simulink model "example_NMPC_BGLOSA_redTh_V500_platoon"  (R2022b)
settings: Solver=ode4  StartTime=0.0  StopTime=1500  FixedStep=0.1  RelTol=1e-3
PostLoadFcn:
  | , if any(exist('dsrtsu_mdlpostloadfcn', 'file') == [2, 3, 6]), try dsrtsu_mdlpostloadfcn('Execute', bdroot); catch fprintf('Error in PostLoadFcn (dsrtsu_mdlpostloadfcn) for model "%s":\n %s\n', bdroot, lasterr); end, end,
values from neighbouring files (symbols this model uses):
  k_road_map = k_road_map(:)    [NMPC_init.m]
  N = 50    [ACADO_BGLOSA_soft_constraints_platoon.m]    (also in ACADO_BGLOSA_soft_constraints_platoon_stop_dwell.m; NMPC_init.m)
  N_iter = 3    [NMPC_init.m]
  N_Jterms = length(Qx1)    [NMPC_init.m]
  NMPC_Wmat1 = [W1(1,:) W1(2,:) W1(3,:) W1(4,:) W1(5,:) W1(6,:) W1(7,:) W1(8,:) W1(9,:)]    [NMPC_init.m]
  NMPC_WNmat1 = reshape(WN1.',1,[])    [NMPC_init.m]
  t_dwell = 10    [ACADO_BGLOSA_soft_constraints_platoon.m]    (also in ACADO_BGLOSA_soft_constraints_platoon_stop_dwell.m; NMPC_init.m)
  t_offset = 0    [NMPC_init.m]
  time_bag_sim = (0:1:round(time_bag(end))-1)'    [NMPC_init.m]
  tl_state_sim = zeros(round(time_bag(end))-1,size(tl_col,2))    [NMPC_init.m]
  Ts = 1    [ACADO_BGLOSA_soft_constraints_platoon.m]    (also in ACADO_BGLOSA_soft_constraints_platoon_stop_dwell.m; NMPC_init.m)
  Vmax = 50    [NMPC_init.m]
  xInit = [0 2 0]    [NMPC_init.m]
undefined symbols (not defined in the file or in its folder): ds, s_start
libraries: simulink x1
(part 1 of 2)
settings Model: DSRTSU_INTERNAL_RTI_VER=450  DSRTSU_INTERNAL_RTI_TYPE=rti1401  DSRTSU_INTERNAL_RTIFPGA=40  Creator=d068515  LastModifiedBy=ricca
settings DataIOCC: SaveFormat=StructureWithTime
settings OptimizationCC: BlockReduction=off  LifeSpan=inf
settings DebuggingCC: SFExecutionAtInitializationDiag=none  SFMachineParentedDataDiag=warning  ArithmeticOperatorsInVariantConditions=warning
settings HardwareCC: ProdBitPerSizeT=32  ProdBitPerPtrDiffT=32  ProdEndianess=BigEndian  ProdWordSize=32  ProdHWDeviceType=Generic->Custom  TargetIntDivRoundTo=Zero  TargetEndianess=BigEndian  TargetHWDeviceType=Generic->Custom
settings SFSimCC: CustomCodeUndefinedFunction=UseInterfaceOnly
settings RTWCC: Description=dSPACE DS1401 Hardware Platform  SystemTargetFile=rti1401.tlc  MakeCommand=make_rti  TemplateMakefile=rti1401.tmf
settings CodeAppCC: StateflowObjectComments=on
settings STFCustomTargetCC: ParMdlRefBuildCompliant=on  GRTInterface=on  SystemTargetFile=rti1401.tlc
settings GRTTargetCC: TargetLangStandard=C89/C90 (ANSI)  CompOptLevelCompliant=off  ConcurrentExecutionCompliant=off  CombineOutputUpdateFcns=off  MatFileLogging=off  CPPClassGenCompliant=off  GRTInterface=on  UseToolchainInfoCompliant=off  ExtModeMexFile=noextcomm

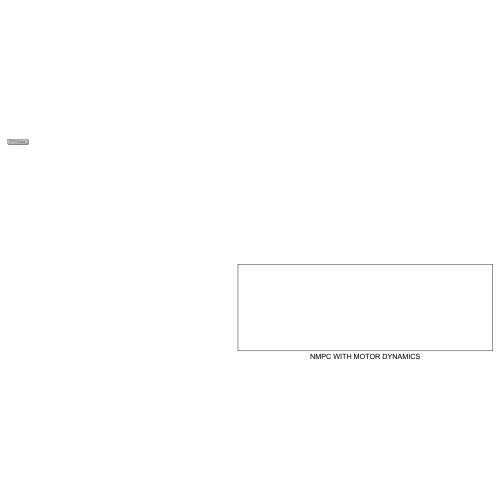
[thumbnail: Simulink's stored preview of the top-level diagram]
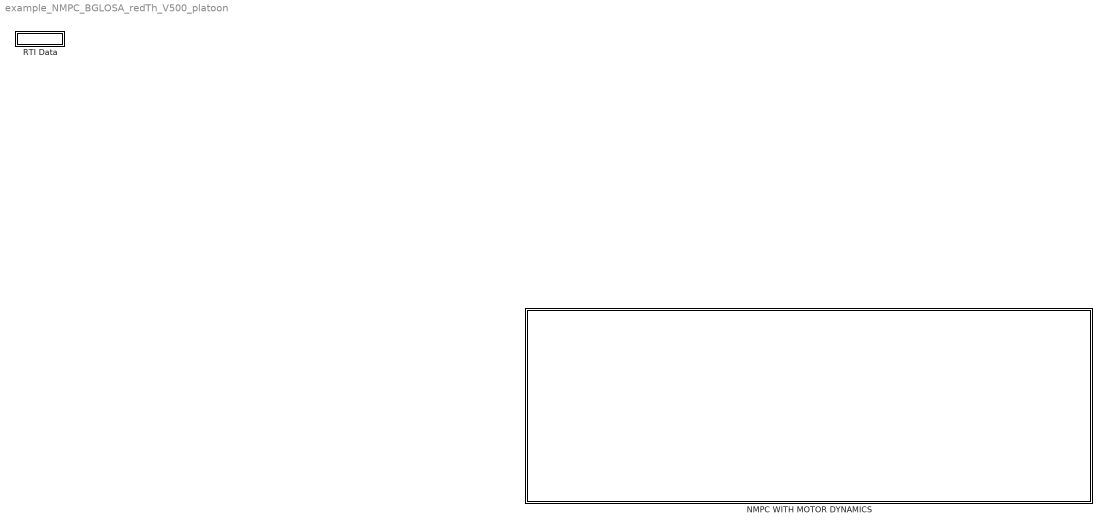
== system example_NMPC_BGLOSA_redTh_V500_platoon ==
  NMPC WITH MOTOR DYNAMICS : Subsystem
  RTI Data : Subsystem  Tag=struct('RTIDataServer',struct('RTIDataServerVs','2','RTIModelDescription','struct(''main'',''TC_RAF_2014b'',''sub'','''',''isMp'',0)'))  LoadFcn="if exist('rtidc'), try,  rtidc('DataHostBlockClbLoad', gcbh); catch, disp(['Warning: ''LoadFcn'' for RTI Data block failed: ' lasterr]); end, end,"  mask(RTI_DATA_HOST){}
      mask help:
      | RTI Data Block.
      | This block is used by RTI to store internal model-dependent data.
      | Please keep this block on the root level of the model. Deleting this block will result in data loss.
      |
      | NEVER DELETE OR COPY THIS BLOCK!
      settings: CopyFcn="if exist('rtidc'), try,  rtidc('DataHostBlockClbCopy', gcbh); catch, disp(['Warning: ''CopyFcn'' for RTI Data block failed: ' lasterr]); end, end,"  DeleteFcn="if exist('rtidc'), try,  rtidc('DataHostBlockClbDelete', gcbh); catch, disp(['Warning: ''DeleteFcn'' for RTI Data block failed: ' lasterr]); end, end,"  ModelCloseFcn="if exist('rtidc'), try,  rtidc('DataHostBlockClbModelClose', gcbh); catch, disp(['Warning: ''ModelCloseFcn'' for RTI Data block failed: ' lasterr]); end, end,"  PreSaveFcn="if exist('rtidc'), try,  rtidc('DataHostBlockClbPreSave', gcbh); catch, disp(['Warning: ''PreSaveFcn'' for RTI Data block failed: ' lasterr]); end, end,"  PostSaveFcn="if exist('rtidc'), try,  rtidc('DataHostBlockClbPostSave', gcbh); catch, disp(['Warning: ''PostSaveFcn'' for RTI Data block failed: ' lasterr]); end, end,"  NameChangeFcn="if exist('rtidc'), try,  rtidc('DataHostBlockClbNameChange', gcbh); catch, disp(['Warning: ''NameChangeFcn'' for RTI Data block failed: ' lasterr]); end, end,"
      mask Help:
      | RTI Data Block.
      | This block is used by RTI to store internal model-dependent data.
      | Please keep this block on the root level of the model. Deleting this block will result in data loss.
      | 
      | NEVER DELETE OR COPY THIS BLOCK!
      mask Display:
      | text(0.5, 0.5, 'RTI Data', 'HorizontalAlignment', 'center');
      | plot([1 0]);

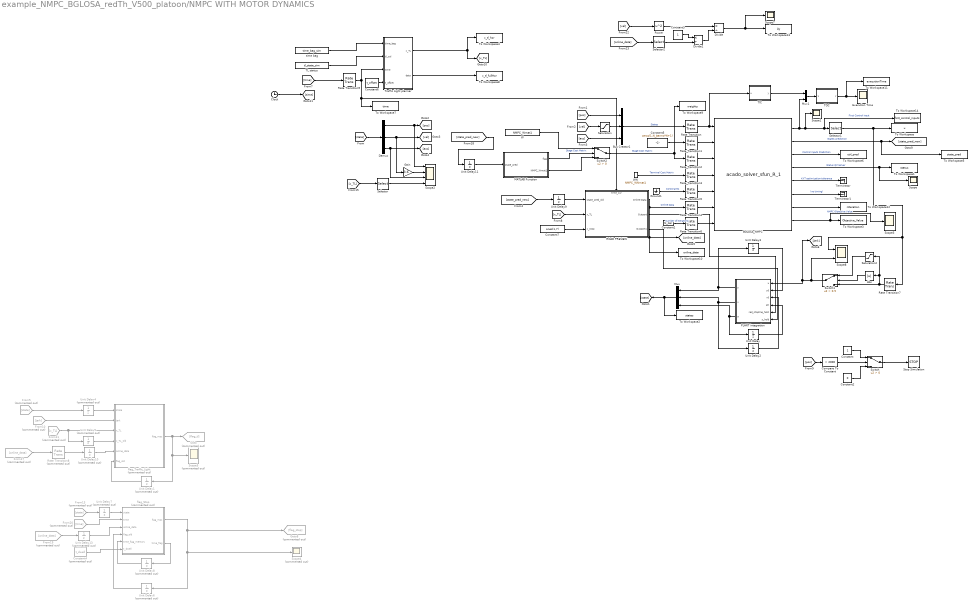
== system example_NMPC_BGLOSA_redTh_V500_platoon/NMPC WITH MOTOR DYNAMICS ==
  Abs : Abs  SaturateOnIntegerOverflow=off
  BGLOSA_NMPC : S-Function  FunctionName=acado_solver_sfun_R_1  Parameters=xInit, zInit, uInit, NMPC_Wmat1, NMPC_WNmat1, bValues  SFunctionDeploymentMode=off  EnableBusSupport=off  mask(Legacy Function){SFunctionSpec=acado_step(ACADOinput u1[1], ACADOoutput y1[1]), ShowSpec=on}
      mask prompts: ShowSpec "Display function specification"
      mask help:
      | This block allows you to call the legacy functions specified by the following Legacy Code Tool definition:
      | def.SFunctionName = 'acado_solver_sfun';
      | def.OutputFcnSpec = 'acado_step(ACADOinput u1[1], ACADOoutput y1[1])';
      | def.StartFcnSpec = 'acado_initialize( void )';
      | def.TerminateFcnSpec = 'acado_cleanup( void )';
      | def.HeaderFiles = {'acado_common.h', 'acado_solver_sfunction.h'};
      | def.SourceFiles = {'acado_solver.c', 'acado_integrator.c', 'acado_auxiliary_functions.c', 'acado_solver_sfunction.c', 'acado_qpoases_interface.cpp', 'qpoases/SRC/Bounds.cpp', 'qpoases/SRC/Constraints.cpp', 'qpoases/SRC/CyclingManager.cpp', 'qpoases/SRC/Indexlist.cpp', 'qpoases/SRC/MessageHandling.cpp', 'qpoases/SRC/QProblem.cpp', 'qpoases/SRC/QProblemB.cpp', 'qpoases/SRC/SubjectTo.cpp', 'qpoases/SRC/Utils.cpp', 'qpoases/SRC/EXTRAS/SolutionAnalysis.cpp'};
      | def.IncPaths = {'qpoases', 'qpoases/INCLUDE', 'qpoases/SRC'};
      | def.Options.language = 'C++';
      mask Help: <p>This block was generated automatically by the Legacy Code Tool. For detailed help on this tool, call<a href="matlab:legacy_code('help')"> legacy_code('help')</a>.</p>
      mask Callback ShowSpec:
      | if strcmp(get_param(gcbh, 'ShowSpec'), 'on')
      |   set_param(gcbh, 'MaskDisplay', sprintf('fprintf(''%s'');', get_param(gcbh, 'SFunctionSpec')));
      | else
      |   set_param(gcbh, 'MaskDisplay', sprintf('fprintf(''%s'');', get_param(gcbh, 'FunctionName')));
      | end
      mask Display: fprintf('acado_step(ACADOinput u1[1], ACADOoutput y1[1])');
  Bus Creator1 : BusCreator  Inputs=3
  Clock : Clock
  Compare To Constant : simulink/Logic and Bit Operations/Compare To Constant  relop=>  const=2000  OutDataTypeStr=boolean
  Constant : Constant
  Constant1 : Constant  Value=N_iter
  Constant2 : Constant  Value=0
  Constant3 : Constant
  Constant4 : Constant  Commented=on  Value=t_dwell
  Constant5 : Constant  Value=zeros(1,N_Jterms*N+1)
  Constant6 : Constant  Value=t_offset
  Constant7 : Constant  Value=ones(1,7)
  Demux : Demux  Outputs=3
  Divide : Product  Inputs=*/
  Divide1 : Product  Inputs=*/
  Execution Time : Scope
  From10 : From  Commented=on  GotoTag=jerk
  From11 : From  Commented=on  GotoTag=x_TL
  From13 : From  Commented=on  GotoTag=state
  From17 : From  Commented=on  GotoTag=online_data
  From19 : From  Commented=on  GotoTag=online_data
  From20 : From  Commented=on  GotoTag=time
  From5 : From  Commented=on  GotoTag=state
  Gain : Gain  Gain=3.6
  Goto : Goto  Commented=on  GotoTag=flag_tl
  Goto8 : Goto  Commented=on  GotoTag=flag_stop
  Ground1 : Ground
  MATLAB Function : MATLAB Function  TreatAsAtomicUnit=on
  Mux : Mux  Inputs=3
  Mux1 : Mux  Inputs=2
  PLANT integration : MATLAB Function  TreatAsAtomicUnit=on
  Power : Math  Operator=square
  ROAD PREVIEW : Subsystem
      settings: PortSchema="{\"entries\":[{\"content\":{\"sides\":[{\"content\":{\"connectorIds\":[\"In1\",\"In2\",\"In3\"]},\"type\":\"ConnectorPlacement.EquallySpacedRectSide\",\"uuid\":\"89746bc5-bd2f-4e61-9556-28242176c46a\"},{\"content\":{\"connectorIds\":[\"Out1\",\"Out2\",\"Out3\"],\"side\":\"RIGHT\"},\"type\":\"ConnectorPlacement.EquallySpacedRectSide\",\"uuid\":\"fa5eae8e-eb55-42b4-8d8b-02c8b36cc91d\"},{\"content\":{\"connectorIds\":[\"In4\"],\"side\":\"TOP\"},\"type\":\"ConnectorPlacement.EquallySpacedRectSide\",\"uuid\":\"5942e98b-dfb5-4e56-acd3-edfb2315bb7f\"}]},\"type\":\"ConnectorPlacement.EquallySpacedConnector\",\"uuid\":\"ba8f73d0-227f-4198-ac0b-e11b2a073141\"}],\"packageUris\":[\"http://schema.mathworks.com/mf0/Connector/R2020b\"],\"version\":\"1.0\"}"
  Rate Transition : RateTransition  Deterministic=off  InitialCondition=xInit  OutPortSampleTime=Ts
  Rate Transition{1..6} (6 alike) : RateTransition  Deterministic=off  OutPortSampleTime=Ts
  Rate Transition7 : RateTransition  Deterministic=off  OutPortSampleTime=0.1
  Rate Transition8 : RateTransition  Commented=on  InitialCondition=zeros(1665,1)  OutPortSampleTime=Ts
  Rate Transition9 : RateTransition  OutPortSampleTime=Ts
  Saturation : Saturate  UpperLimit=50/3.6  LowerLimit=0
  Saturation2 : Saturate  UpperLimit=0.1  LowerLimit=-0.1
  Scope{,1,3,7} (4 alike) : Scope
  Scope2 : Scope  NumInputPorts=4
  Scope4 : Scope  Commented=on
  Scope5 : Scope  Commented=on
  Scope8 : Scope  NumInputPorts=2
  Selector : Selector  NumberOfDimensions=2  InputPortWidth=3  IndexOptions=Index vector (dialog),Select all  Indices=1,1  OutputSizes=1,1
  Selector1 : Selector  InputPortWidth=3  IndexOptions=Index vector (dialog)  Indices=[1]  OutputSizes=1
  Selector2 : Selector  NumberOfDimensions=2  InputPortWidth=3  IndexOptions=Select all,Select all  Indices=28,1  OutputSizes=1,1
  Stop Simulation : Stop
  Switch : Switch  Criteria=u2 > Threshold  SaturateOnIntegerOverflow=off  InputSameDT=off
  Switch1 : Switch  Criteria=u2 > Threshold  Threshold=0.5  SaturateOnIntegerOverflow=off  InputSameDT=off
  Switch2 : Switch  Criteria=u2 > Threshold  SaturateOnIntegerOverflow=off  InputSameDT=off
  TIC : MATLAB Function  TreatAsAtomicUnit=on
  TL status : Constant  Value=tl_state_sim  OutDataTypeStr=double
  TOC : MATLAB Function  TreatAsAtomicUnit=on
  Terminator : Terminator
  Terminator1 : Terminator
  To Workspace : ToWorkspace  VariableName=u  SaveFormat=Structure With Time  SampleTime=-1
  To Workspace1 : ToWorkspace  VariableName=status  SaveFormat=Structure With Time  SampleTime=-1
  To Workspace10 : ToWorkspace  VariableName=online_data  SaveFormat=Structure With Time  SampleTime=-1
  To Workspace11 : ToWorkspace  VariableName=executionTime  SaveFormat=Structure With Time  SampleTime=-1
  To Workspace12 : ToWorkspace  VariableName=nIteration  SaveFormat=Structure With Time  SampleTime=-1
  To Workspace13 : ToWorkspace  VariableName=Ay  SaveFormat=Structure With Time  SampleTime=-1
  To Workspace14 : ToWorkspace  VariableName=first_control_inputs  SaveFormat=Timeseries  SampleTime=-1
  To Workspace2 : ToWorkspace  VariableName=states  SaveFormat=Structure With Time  SampleTime=-1
  To Workspace3 : ToWorkspace  VariableName=Objective_Value  SaveFormat=Structure With Time  SampleTime=-1
  To Workspace4 : ToWorkspace  VariableName=x_tl_hor  SaveFormat=Structure With Time  SampleTime=-1
  To Workspace5 : ToWorkspace  VariableName=state_pred  SaveFormat=Structure With Time  SampleTime=-1
  To Workspace6 : ToWorkspace  VariableName=ctrl_pred  SaveFormat=Structure With Time  SampleTime=-1
  To Workspace7 : ToWorkspace  VariableName=time  SaveFormat=Structure With Time  SampleTime=-1
  To Workspace8 : ToWorkspace  VariableName=x_tl_fullHor  SaveFormat=Structure With Time  SampleTime=-1
  To Workspace9 : ToWorkspace  VariableName=weights  SaveFormat=Structure With Time  SampleTime=-1
  Traffic Light planner : MATLAB Function  TreatAsAtomicUnit=on
  Unit Delay : UnitDelay  InitialCondition=xInit(3)  SampleTime=-1  HasFrameUpgradeWarning=on
  Unit Delay1 : UnitDelay  Commented=on  InitialCondition=zeros(1,11)  SampleTime=-1  HasFrameUpgradeWarning=on
  Unit Delay10 : UnitDelay  Commented=on  InitialCondition=zeros(50*(N+1),1)  SampleTime=-1  HasFrameUpgradeWarning=on
  Unit Delay11 : UnitDelay  InitialCondition=xInit.*ones(N+1,3)  SampleTime=-1  HasFrameUpgradeWarning=on
  Unit Delay13 : UnitDelay  Commented=on  InitialCondition=zeros(50*(N+1),1)  SampleTime=-1  HasFrameUpgradeWarning=on
  Unit Delay2 : UnitDelay  InitialCondition=xInit(2)  SampleTime=-1  HasFrameUpgradeWarning=on
  Unit Delay3 : UnitDelay  InitialCondition=xInit(1)  SampleTime=-1  HasFrameUpgradeWarning=on
  Unit Delay4 : UnitDelay  Commented=on  InitialCondition=xInit  SampleTime=-1  HasFrameUpgradeWarning=on
  Unit Delay5 : UnitDelay  Commented=on  InitialCondition=zeros(N+1,12)  SampleTime=-1  HasFrameUpgradeWarning=on
  Unit Delay6 : UnitDelay  Commented=on  InitialCondition=zeros(1,7)  SampleTime=-1  HasFrameUpgradeWarning=on
  Unit Delay7 : UnitDelay  Commented=on  InitialCondition=xInit  SampleTime=-1  HasFrameUpgradeWarning=on
  Unit Delay8 : UnitDelay  Commented=on  InitialCondition=zeros(1,7)  SampleTime=-1  HasFrameUpgradeWarning=on
  Unit Delay9 : UnitDelay  InitialCondition=xInit.*ones(N+1,3)  SampleTime=-1  HasFrameUpgradeWarning=on
  W : Constant  Value=NMPC_Wmat1  OutDataTypeStr=double
  "WN " : Constant  Value=NMPC_WNmat1  OutDataTypeStr=double
  flag_Stop : MATLAB Function  Commented=on  TreatAsAtomicUnit=on
  flag_Traffic_Light : MATLAB Function  Commented=on  TreatAsAtomicUnit=on
  time bag : Constant  Value=time_bag_sim  OutDataTypeStr=double
  wires:
  BGLOSA_NMPC/3 -> To Workspace6/1  "Control Inputs Prediction"
  BGLOSA_NMPC/4 -> To Workspace1/1, Scope/1  "Status QP Solver"
  Constant1/1 -> Rate Transition6/1  "Number of iterations"
  BGLOSA_NMPC/8 -> Scope3/1, To Workspace3/1  "NMPC Objective Value"
  Bus Creator1/1 -> Rate Transition/1  "States"
  BGLOSA_NMPC/1 -> Mux1/2, To Workspace14/1, Selector1/1, Scope1/1  "First Control Input"
  BGLOSA_NMPC/5 -> Terminator/1  "KKT optimization tolerance"
  BGLOSA_NMPC/6 -> Terminator1/1  "(no timing)"
  Ground1/1 -> Rate Transition5/1  "Constraints"
  BGLOSA_NMPC/7 -> To Workspace12/1
  Rate Transition1/1 -> BGLOSA_NMPC/2
  Rate Transition2/1 -> BGLOSA_NMPC/3
  Rate Transition6/1 -> BGLOSA_NMPC/7
  Rate Transition3/1 -> BGLOSA_NMPC/4
  Rate Transition5/1 -> BGLOSA_NMPC/5
  Rate Transition4/1 -> BGLOSA_NMPC/6
  BGLOSA_NMPC/2 -> To Workspace5/1, [state_pred_new]  "States prediction"
  Constant5/1 -> Rate Transition1/1
  Demux/1 -> Scope2/1, [pos]
  Demux/2 -> [vel], Gain/1
  Demux/3 -> Scope2/3, [acc]
  PLANT integration/2(v) -> Mux/2, Unit Delay2/1
  PLANT integration/1(s) -> Unit Delay3/1, Mux/1
  PLANT integration/3(a) -> Mux/3, Unit Delay/1
  Unit Delay3/1 -> PLANT integration/2(s0)
  ROAD PREVIEW/1(Online Data) -> [online_data], To Workspace10/1, Rate Transition4/1  "Online Data"
  Switch2/1 -> Rate Transition2/1, To Workspace9/1  "Stage Cost Matrix"
  "WN "/1 -> Rate Transition3/1  "Terminal Cost Matrix"
  Selector1/1 -> Rate Transition7/1, Scope8/1, To Workspace/1
  Unit Delay/1 -> PLANT integration/4(a0)
  Unit Delay2/1 -> PLANT integration/3(v0)
  Mux/1 -> To Workspace2/1, [state]
  [state] -> Demux/1
  [pos] -> Bus Creator1/1
  [vel] -> Saturation/1
  [acc] -> Bus Creator1/3
  [state_pred_new] -> Unit Delay9/1
  From5/1 -> Unit Delay4/1
  From10/1 -> flag_Traffic_Light/2(jerk)
  [x_TL] -> ROAD PREVIEW/2(x_TL)
  From11/1 -> flag_Traffic_Light/3(x_TL), Unit Delay5/1
  flag_Traffic_Light/1(flag_mpc) -> Unit Delay1/1, Scope5/1, Goto/1
  Unit Delay1/1 -> flag_Traffic_Light/6(flag_old)
  Unit Delay4/1 -> flag_Traffic_Light/1(state)
  Unit Delay5/1 -> flag_Traffic_Light/4(x_TL_old)
  Unit Delay7/1 -> flag_Stop/1(state)
  Unit Delay6/1 -> flag_Stop/4(flag_old)
  flag_Stop/1(flag_mpc) -> Goto8/1, Unit Delay6/1, Scope4/1
  From20/1 -> flag_Stop/2(time)
  From13/1 -> Unit Delay7/1
  Constant7/1 -> ROAD PREVIEW/3(x_stop)
  Unit Delay9/1 -> ROAD PREVIEW/1(state_pred_old)
  time bag/1 -> Traffic Light planner/1(time_bag)
  TL status/1 -> Traffic Light planner/2(tl_col)
  Rate Transition9/1 -> ROAD PREVIEW/4(time_cur), To Workspace7/1, Traffic Light planner/3(time)
  [x_TL] -> Selector/1
  From17/1 -> Rate Transition8/1
  Unit Delay10/1 -> flag_Traffic_Light/5(online_data)
  Selector/1 -> Scope2/4
  flag_Stop/2(time_flag) -> Unit Delay8/1
  Unit Delay8/1 -> flag_Stop/5(time_flag_memory)
  Saturation/1 -> Bus Creator1/2
  [pos] -> Compare To Constant/1
  Compare To Constant/1 -> Switch/2
  Constant/1 -> Switch/1
  Constant2/1 -> Switch/3
  Switch/1 -> Stop Simulation/1
  Rate Transition8/1 -> Unit Delay10/1
  From19/1 -> Unit Delay13/1
  Unit Delay13/1 -> flag_Stop/3(online_data)
  Switch1/1 -> Scope8/2, [jerk], PLANT integration/1(u)
  Rate Transition7/1 -> Saturation2/1, Abs/1, Switch1/3
  Abs/1 -> Switch1/2
  Saturation2/1 -> Switch1/1
  Gain/1 -> Scope2/2
  Power/1 -> Divide/1
  Divide1/1 -> Divide/2
  [vel] -> Power/1
  Constant3/1 -> Divide1/1
  [online_data] -> Selector2/1
  Selector2/1 -> Divide1/2
  Divide/1 -> Scope7/1, To Workspace13/1
  Constant4/1 -> flag_Stop/6(t_dwell)
  [time] -> Rate Transition9/1
  Constant6/1 -> Traffic Light planner/4(t_offset)
  TOC/1(y) -> To Workspace11/1, Execution Time/1
  Rate Transition/1 -> TIC/1(u), BGLOSA_NMPC/1
  Mux1/1 -> TOC/1(u)
  TIC/1(y) -> Mux1/1
  W/1 -> Switch2/1  "Stage Cost Matrix"
  [state_pred_new] -> Unit Delay11/1
  Unit Delay11/1 -> MATLAB Function/1(state_pred)
  MATLAB Function/1(flag) -> Switch2/2
  MATLAB Function/2(NMPC_Wmat1) -> Switch2/3
  Traffic Light planner/1(x_TL) -> [x_TL], To Workspace4/1
  Traffic Light planner/2(data) -> To Workspace8/1
  Clock/1 -> [time]
  ROAD PREVIEW/2(Outport) -> PLANT integration/5(red_stopline_hold)
  ROAD PREVIEW/3(Outport1) -> PLANT integration/6(s_hold)

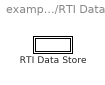
== system example_NMPC_BGLOSA_redTh_V500_platoon/RTI Data ==
  RTI Data Store : Subsystem  Tag="struct('private',struct('version',struct('dsVer',uint32(2),'dsVerCreation',uint32(2),'RTI',struct('ver','7.3','type','RTI1401')),'access',struct('type','Model','isPerm',1,'created',['23-Jan-2024 14:08:40'],'modified',['23-Jan-2024 15:26:34'],'location','')),'public',struct('main',struct('data',[]),'sub',struct('name',{{'TC_RAF_2014b'}},'data',{{struct('TH',struct('thTaskInfo',struct('taskType',{'TIMER','HWINT','TMRINT','SWINT','GLINT'},'tasksNumOf',{1,0,0,0,0},'srcIds',{{'TIMERA'},{},{},{},{}},'taskNames',{{['Timer Task 1']},{},{},{},{}})),'th_tc',struct('dataType','TASK','taskGroupId','','taskGroupList',{{}},'taskSchedulingPolicy','FCFS','taskType','TIMER','blkh',-1,'srcId','TIMERA','srcSgnName',['Timer A interrupt'],'srcCpuName','','taskName',['Timer Task 1  [0.01] s'],'taskNameDisplayExt','','smplTime',0.01,'smplTimeOffs',0,'hasFixedPriority',0,'priority',1,'hasFixedOvc',0,'ovcType',1,'ovcMax',1),'tc_th',struct('dataType','TASK','taskGroupId','','taskGroupList',{{}},'taskSchedulingPolicy','FCFS','taskType','TIMER','blkh',-1,'srcId','TIMERA','srcSgnName',['Timer A interrupt'],'srcCpuName','','taskName',['Timer Task 1  [0.01] s'],'taskNameDisplayExt','','smplTime',0.01,'smplTimeOffs',0,'hasFixedPriority',0,'priority',1,'hasFixedOvc',0,'ovcType',1,'ovcMax',1))}})))"  mask(RTI_DATA_STORE){}
      mask help:
      | RTI Data Store Block. This block is used by RTI to store internal model dependent data. Deleting this block will result in data loss.
      |
      | NEVER DELETE, COPY, OR MODIFY THIS BLOCK!
      mask Help:
      | RTI Data Store Block. This block is used by RTI to store internal model dependent data. Deleting this block will result in data loss.
      | 
      | NEVER DELETE, COPY, OR MODIFY THIS BLOCK!
      mask Display: text(0.5, 0.5, ' ', 'HorizontalAlignment', 'center');

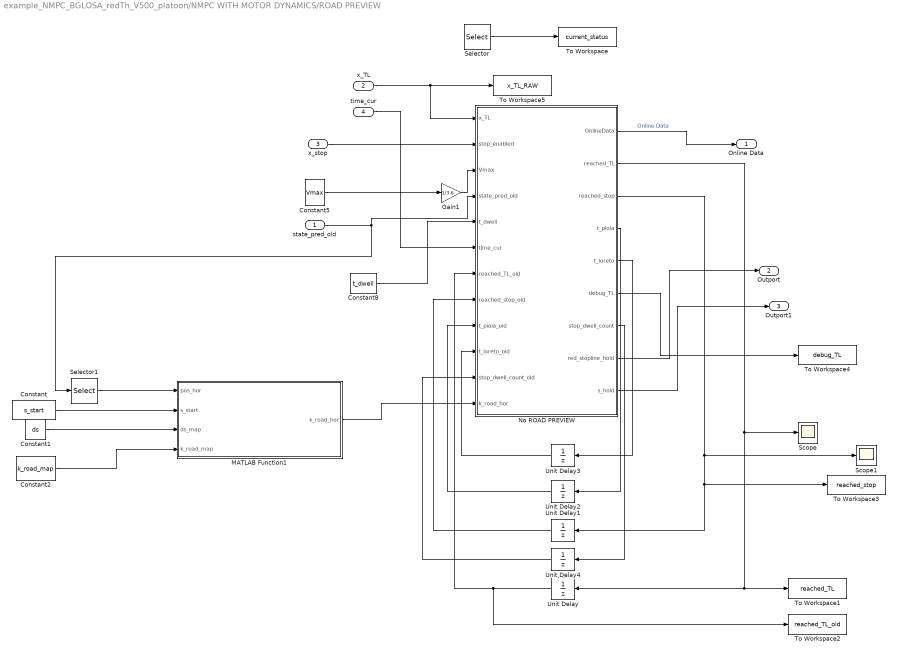
== system example_NMPC_BGLOSA_redTh_V500_platoon/NMPC WITH MOTOR DYNAMICS/ROAD PREVIEW ==
  state_pred_old : Inport
  x_TL : Inport  Port=2
  x_stop : Inport  Port=3
  time_cur : Inport  Port=4
  Constant : Constant  Value=s_start
  Constant1 : Constant  Value=ds
  Constant2 : Constant  Value=k_road_map
  Constant5 : Constant  Value=Vmax
  Constant8 : Constant  Value=t_dwell  VectorParams1D=off
  Gain1 : Gain  Gain=1/3.6
  MATLAB Function1 : MATLAB Function  TreatAsAtomicUnit=on
  No ROAD PREVIEW : MATLAB Function  TreatAsAtomicUnit=on  SystemSampleTime=Ts
  Scope : Scope
  Scope1 : Scope
  Selector : Selector  NumberOfDimensions=2  InputPortWidth=3  IndexOptions=Index vector (dialog),Select all  Indices=1,1  OutputSizes=1,1
  Selector1 : Selector  NumberOfDimensions=2  InputPortWidth=3  IndexOptions=Select all,Index vector (dialog)  Indices=[1 3],1  OutputSizes=1,1
  To Workspace : ToWorkspace  VariableName=current_status  SaveFormat=Structure With Time  SampleTime=-1
  To Workspace1 : ToWorkspace  VariableName=reached_TL  SaveFormat=Structure With Time  SampleTime=-1
  To Workspace2 : ToWorkspace  VariableName=reached_TL_old  SaveFormat=Structure With Time  SampleTime=-1
  To Workspace3 : ToWorkspace  VariableName=reached_stop  SaveFormat=Structure With Time  SampleTime=-1
  To Workspace4 : ToWorkspace  VariableName=debug_TL  SaveFormat=Timeseries  SampleTime=-1
  To Workspace5 : ToWorkspace  VariableName=x_TL_RAW  SaveFormat=Timeseries  SampleTime=-1
  Unit Delay : UnitDelay  InitialCondition=zeros(1,11)  SampleTime=-1  HasFrameUpgradeWarning=on
  Unit Delay1 : UnitDelay  InitialCondition=zeros(1,7)  SampleTime=-1  HasFrameUpgradeWarning=on
  Unit Delay2 : UnitDelay  SampleTime=-1  HasFrameUpgradeWarning=on
  Unit Delay3 : UnitDelay  SampleTime=-1  HasFrameUpgradeWarning=on
  Unit Delay4 : UnitDelay  InitialCondition=zeros(1,7)  SampleTime=-1  HasFrameUpgradeWarning=on
  Online Data : Outport
  Outport : Outport  Port=2
  Outport1 : Outport  Port=3
  wires:
  No ROAD PREVIEW/1(OnlineData) -> Online Data/1  "Online Data"
  Constant5/1 -> Gain1/1
  Gain1/1 -> No ROAD PREVIEW/3(Vmax)
  state_pred_old/1 -> Selector1/1, No ROAD PREVIEW/4(state_pred_old)
  Selector/1 -> To Workspace/1
  No ROAD PREVIEW/2(reached_TL) -> To Workspace1/1, Unit Delay/1, Scope/1
  Unit Delay/1 -> No ROAD PREVIEW/7(reached_TL_old), To Workspace2/1
  x_TL/1 -> No ROAD PREVIEW/1(x_TL), To Workspace5/1
  x_stop/1 -> No ROAD PREVIEW/2(stop_enabled)
  No ROAD PREVIEW/3(reached_stop) -> To Workspace3/1, Unit Delay1/1, Scope1/1
  Unit Delay1/1 -> No ROAD PREVIEW/8(reached_stop_old)
  Constant8/1 -> No ROAD PREVIEW/5(t_dwell)
  No ROAD PREVIEW/4(t_piola) -> Unit Delay2/1
  No ROAD PREVIEW/5(t_loreto) -> Unit Delay3/1
  Unit Delay2/1 -> No ROAD PREVIEW/9(t_piola_old)
  Unit Delay3/1 -> No ROAD PREVIEW/10(t_loreto_old)
  No ROAD PREVIEW/6(debug_TL) -> To Workspace4/1
  Unit Delay4/1 -> No ROAD PREVIEW/11(stop_dwell_count_old)
  No ROAD PREVIEW/7(stop_dwell_count) -> Unit Delay4/1
  No ROAD PREVIEW/8(red_stopline_hold) -> Outport/1
  No ROAD PREVIEW/9(s_hold) -> Outport1/1
  Constant2/1 -> MATLAB Function1/4(k_road_map)
  Constant1/1 -> MATLAB Function1/3(ds_map)
  Constant/1 -> MATLAB Function1/2(s_start)
  MATLAB Function1/1(k_road_hor) -> No ROAD PREVIEW/12(k_road_hor)
  Selector1/1 -> MATLAB Function1/1(pos_hor)
  time_cur/1 -> No ROAD PREVIEW/6(time_cur)

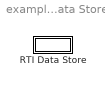
== system example_NMPC_BGLOSA_redTh_V500_platoon/RTI Data/RTI Data Store ==
  RTI Data Store : Subsystem  mask(RTI_DATA_STORE){}
      mask help:
      | RTI Data Store Block. This block is used by RTI to store internal model dependent data. Deleting this block will result in data loss.
      |
      | NEVER DELETE, COPY, OR MODIFY THIS BLOCK!
      mask Help:
      | RTI Data Store Block. This block is used by RTI to store internal model dependent data. Deleting this block will result in data loss.
      | 
      | NEVER DELETE, COPY, OR MODIFY THIS BLOCK!
      mask Display: text(0.5, 0.5, ' ', 'HorizontalAlignment', 'center');

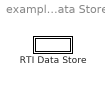
== system example_NMPC_BGLOSA_redTh_V500_platoon/RTI Data/RTI Data Store/RTI Data Store ==
  RTI Data Store : Subsystem  mask(RTI_DATA_STORE){}
      mask help:
      | RTI Data Store Block. This block is used by RTI to store internal model dependent data. Deleting this block will result in data loss.
      |
      | NEVER DELETE, COPY, OR MODIFY THIS BLOCK!
      mask Help:
      | RTI Data Store Block. This block is used by RTI to store internal model dependent data. Deleting this block will result in data loss.
      | 
      | NEVER DELETE, COPY, OR MODIFY THIS BLOCK!
      mask Display: text(0.5, 0.5, ' ', 'HorizontalAlignment', 'center');

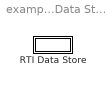
== system example_NMPC_BGLOSA_redTh_V500_platoon/RTI Data/RTI Data Store/RTI Data Store/RTI Data Store ==
  RTI Data Store : Subsystem  mask(RTI_DATA_STORE){}
      mask help:
      | RTI Data Store Block. This block is used by RTI to store internal model dependent data. Deleting this block will result in data loss.
      |
      | NEVER DELETE, COPY, OR MODIFY THIS BLOCK!
      mask Help:
      | RTI Data Store Block. This block is used by RTI to store internal model dependent data. Deleting this block will result in data loss.
      | 
      | NEVER DELETE, COPY, OR MODIFY THIS BLOCK!
      mask Display: text(0.5, 0.5, ' ', 'HorizontalAlignment', 'center');

== system example_NMPC_BGLOSA_redTh_V500_platoon/RTI Data/RTI Data Store/RTI Data Store/RTI Data Store/RTI Data Store ==

== matlab function example_NMPC_BGLOSA_redTh_V500_platoon/NMPC WITH MOTOR DYNAMICS/PLANT integration ==
  data: s output; v output; a output; u input; s0 input; v0 input; a0 input; red_stopline_hold input; s_hold input
function [s, v, a] = plant_integrator(u, s0, v0, a0, red_stopline_hold, s_hold)

dt = 0.1;

if red_stopline_hold
    s = min(s0, s_hold);
    v = 0;
    a = 0;
    return
end

% ============================================================
% INTEGRAZIONE NORMALE
% ============================================================

Ax_min = -1.5;
Ax_max =  1.5;

a = a0 + u*dt;

if a > Ax_max
    a = Ax_max;
elseif a < Ax_min
    a = Ax_min;
end

v = v0 + a*dt;

if v < 0
    v = 0;
end

s = s0 + v*dt;

end

== matlab function example_NMPC_BGLOSA_redTh_V500_platoon/NMPC WITH MOTOR DYNAMICS/flag_Traffic_Light ==
  data: state input; jerk input; x_TL input; x_TL_old input; online_data input; flag_old input; flag_mpc output
function flag_mpc = fcn(state, jerk, x_TL, x_TL_old, online_data, flag_old)

s_TL = [45.5, 203.2, 384.2, 589.4, 773.6, 1004.2, ...
        1225.3, 1419.7, 1507.8, 1739.0, 1823.0];

s_max = 5200;
N = 50;
N_od = 50;
N_TL = 11;

flag_mpc = zeros(1,N_TL);
flag_old = flag_old(:).';

for ii = 1:N_TL

    x_now = x_TL(1,ii);
    x_old = x_TL_old(1,ii);

    if x_now == x_old
        flag_old(1,ii) = flag_old(1,ii);
    else
        flag_old(1,ii) = 0;
    end

    if x_now == 0
        if state(2) < 0.1 && abs(s_TL(ii) - state(1)) < 0.5
            flag_mpc(1,ii) = 1;
        else
            flag_mpc(1,ii) = 0;
        end
    else
        if abs(s_max - state(1)) < 0.5 && flag_old(1,ii) == 1
            flag_mpc(1,ii) = 1;
        else
            flag_mpc(1,ii) = 0;
        end
    end

    if state(1) >= s_TL(ii) || sum(online_data(ii:N_od:end)) == N+1
        flag_mpc(1,ii) = 0;
    end

end

== matlab function example_NMPC_BGLOSA_redTh_V500_platoon/NMPC WITH MOTOR DYNAMICS/Traffic Light planner ==
  data: time_bag input; x_TL output size=[51 12]; tl_col input; time input; data output size=[51 12]; t_offset input
function [x_TL,data] = get_TL_data(time_bag, tl_col, time, t_offset)
%#codegen

N = 50;
n_tl = size(tl_col,2);

x_TL = zeros(N+1,n_tl);
data = zeros(N+1,n_tl);

Ts_ocp  = 1.0;   % passo nodi NMPC [s]
Ts_spat = 1.0;   % passo righe tl_col [s]

n_rows = size(tl_col,1);

% -------------------------------------------------------------------------
% x_TL: preview semaforico usato dal NMPC, con t_offset
% -------------------------------------------------------------------------
for kk = 1:N+1

    t_k = time + t_offset + (kk-1)*Ts_ocp;

    row = floor(t_k/Ts_spat) + 1;
    row = max(1, min(row, n_rows));

    x_TL(kk,:) = tl_col(row,:);

end

% -------------------------------------------------------------------------
% data: preview semaforico senza t_offset, per diagnostica/confronto
% -------------------------------------------------------------------------
for kk = 1:N+1

    t_k = time + (kk-1)*Ts_ocp;

    row = floor(t_k/Ts_spat) + 1;
    row = max(1, min(row, n_rows));

    data(kk,:) = tl_col(row,:);

end

end

== matlab function example_NMPC_BGLOSA_redTh_V500_platoon/NMPC WITH MOTOR DYNAMICS/MATLAB Function ==
  data: flag output; state_pred input; NMPC_Wmat1 output
function [flag, NMPC_Wmat1] = fcn(state_pred)

pos_hor = state_pred(:,1);

if pos_hor(1) > 1500 && pos_hor(1) < 1800
    flag = 0;
else
    flag = 1;
end

Qx1 = [10 2 0.5 10000 10000 50 200 500 100];
W1 = diag(Qx1);
NMPC_Wmat1 = reshape(W1.',1,[]);

== matlab function example_NMPC_BGLOSA_redTh_V500_platoon/NMPC WITH MOTOR DYNAMICS/ROAD PREVIEW/MATLAB Function1 ==
  data: pos_hor input; k_road_hor output; s_start input; ds_map input; k_road_map input
function k_road_hor = RoadCurvaturePreview(pos_hor, s_start, ds_map, k_road_map)

N = 50;
k_road_hor = zeros(N+1,1);

n_map = length(k_road_map);

for kk = 1:N+1

    s_pred = pos_hor(kk);

    eta = (s_pred - s_start)/ds_map + 1;

    idx0 = floor(eta);
    alpha = eta - idx0;

    if idx0 < 1

        k_val = k_road_map(1);

    elseif idx0 >= n_map

        k_val = k_road_map(n_map);

    else

        k0 = k_road_map(idx0);
        k1 = k_road_map(idx0 + 1);

        k_val = k0 + alpha*(k1 - k0);

    end

    if ~isfinite(k_val)
        k_val = 0;
    end

    k_road_hor(kk) = abs(k_val);

end

== matlab function example_NMPC_BGLOSA_redTh_V500_platoon/NMPC WITH MOTOR DYNAMICS/TIC ==
  data: y output; u input
function y = fcn(u)
% The output y is of size 2x1.
%
% Zihao Liu 23/5/2020
% Last Change 23/5/2020

y = zeros(2,1);
t = tic; % During Code Gen, MATLAB returns a struct contains tv_sec and tv_nsec.
y(1) = t.tv_sec;
y(2) = t.tv_nsec;


end

== matlab function example_NMPC_BGLOSA_redTh_V500_platoon/NMPC WITH MOTOR DYNAMICS/TOC ==
  data: u input; y output
function y = fcn(u)
% Output y is a double scaler, in seconds.
%
%
% Zihao Liu 23/5/2020
% Last Change 23/5/2020


% Reconstruct the struct from tic.
t.tv_sec = u(1);
t.tv_nsec = u(2);
y = toc(t);

end
